simulink model "NLsim"  (R2021a)
settings: Solver=FixedStepAuto  StartTime=0.0  StopTime=200  FixedStep=0.01  RelTol=1e-3
undefined symbols (not defined in the file): g, Ixx, Iyy, Izz, m, phi0, psi0, Stability_Matrix, theta0, WD0, X0, X0_Y0_Z0
libraries: shared6dof x1
settings Model: Creator=User01  LastModifiedBy=User01

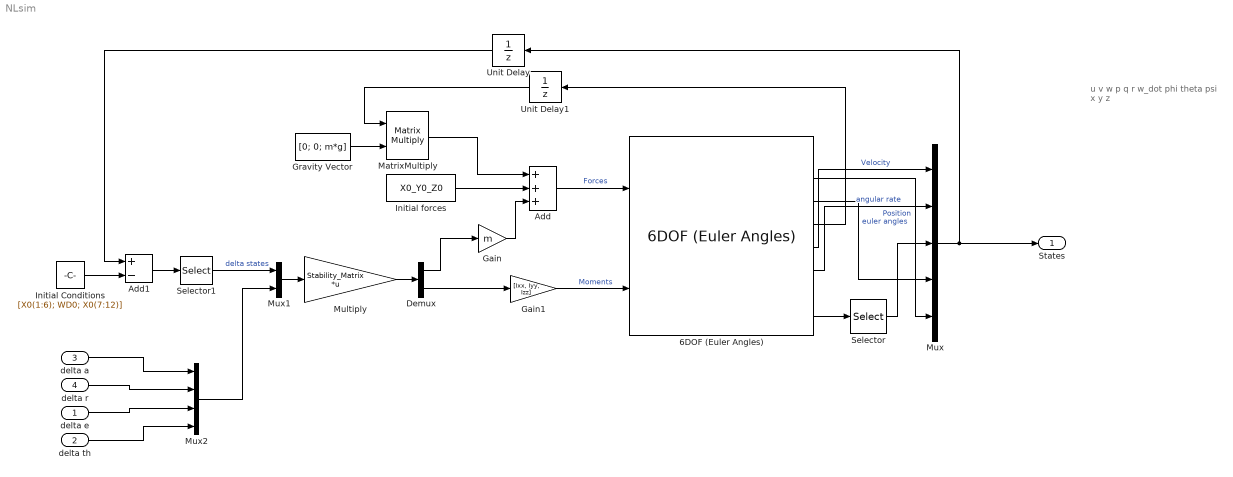
== system NLsim ==
  note: u
      | v
      | w
      |
      | p
      | q
      | r
      |
      | w_dot
      |
      | phi
      | theta
      | psi
      |
      | x
      | y
      | z
  delta e : Inport
  delta th : Inport  Port=2
  delta a : Inport  Port=3
  delta r : Inport  Port=4
  6DOF (Euler Angles) : shared6dof/6DOF (Euler Angles)  units=English (Velocity in ft/s)  mtype=Fixed  rep=Euler Angles  xme_0=X0(10:12)  Vm_0=X0(1:3)  eul_0=X0(7:9)  pm_0=X0(4:6)  mass_0=m  mass_e=0.5  mass_f=2.0  inertia=I  inertia_e=eye(3)  inertia_f=2*eye(3)  k_quat=1.0  vre_flag=on  abi_flag=off  aMode=0  xme_statename=''  Vm_statename=''  eul_statename=''  quat_statename=''  pm_statename=''  mass_statename=''
      settings: SourceProductBaseCode=AE,PW,DR,MT,UV,VE
  Add : Sum  Inputs=+++
  Add1 : Sum  Inputs=+-
  Demux : Demux  Outputs=2
  Gain : Gain  Gain=m
  Gain1 : Gain  Gain=[Ixx, Iyy, Izz]
  Gravity Vector : Constant  Value=[0; 0; m*g]
  Initial Conditions : Constant  Value=[X0(1:6); WD0; X0(7:12)]
  Initial forces : Constant  Value=X0_Y0_Z0
  MatrixMultiply : Product  Multiplication=Matrix(*)
  Multiply : Gain  Gain=Stability_Matrix  Multiplication=Matrix(K*u)
  Mux : Mux  Inputs=5
  Mux1 : Mux  Inputs=2
  Mux2 : Mux
  Selector : Selector  InputPortWidth=3  IndexOptions=Index vector (dialog)  Indices=3  OutputSizes=1
  Selector1 : Selector  InputPortWidth=13  IndexOptions=Index vector (dialog)  Indices=[1:7]  OutputSizes=1
  Unit Delay : UnitDelay  InitialCondition=[X0(1:6); WD0; X0(7:12)]  SampleTime=-1  HasFrameUpgradeWarning=on
  Unit Delay1 : UnitDelay  InitialCondition=angle2dcm(psi0, theta0, phi0)  SampleTime=-1  HasFrameUpgradeWarning=on
  States : Outport
  wires:
  Initial forces/1 -> Add/2
  6DOF (Euler Angles)/4 -> Unit Delay1/1
  6DOF (Euler Angles)/8 -> Selector/1
  6DOF (Euler Angles)/5 -> Mux/1  "Velocity"
  6DOF (Euler Angles)/6 -> Mux/2  "angular rate"
  6DOF (Euler Angles)/3 -> Mux/4  "euler angles"
  6DOF (Euler Angles)/2 -> Mux/5  "Position"
  Selector/1 -> Mux/3
  Add/1 -> 6DOF (Euler Angles)/1  "Forces"
  Gain/1 -> Add/3
  Initial Conditions/1 -> Add1/2
  Mux/1 -> States/1, Unit Delay/1
  Add1/1 -> Selector1/1
  Selector1/1 -> Mux1/1  "delta states"
  Mux1/1 -> Multiply/1
  Mux2/1 -> Mux1/2
  Multiply/1 -> Demux/1
  Demux/1 -> Gain/1
  Gain1/1 -> 6DOF (Euler Angles)/2  "Moments"
  Demux/2 -> Gain1/1
  Gravity Vector/1 -> MatrixMultiply/2
  MatrixMultiply/1 -> Add/1
  Unit Delay/1 -> Add1/1
  Unit Delay1/1 -> MatrixMultiply/1
  delta a/1 -> Mux2/1
  delta r/1 -> Mux2/2
  delta e/1 -> Mux2/3
  delta th/1 -> Mux2/4
